simulink model "SimCoJLinkExample_G071"  (R2020b)
settings: Solver=FixedStepDiscrete  StartTime=0.0  StopTime=inf  RelTol=1e-3
undefined symbols (not defined in the file): Cortex, M4
libraries: SimCoJLink x3
settings Model: Creator=beau_  LastModifiedBy=beau_
settings DataIOCC: SaveOutput=off  SignalLogging=off  DSMLogging=off  SaveTime=off  ReturnWorkspaceOutputs=off
settings DebuggingCC: ParameterPrecisionLossMsg=none

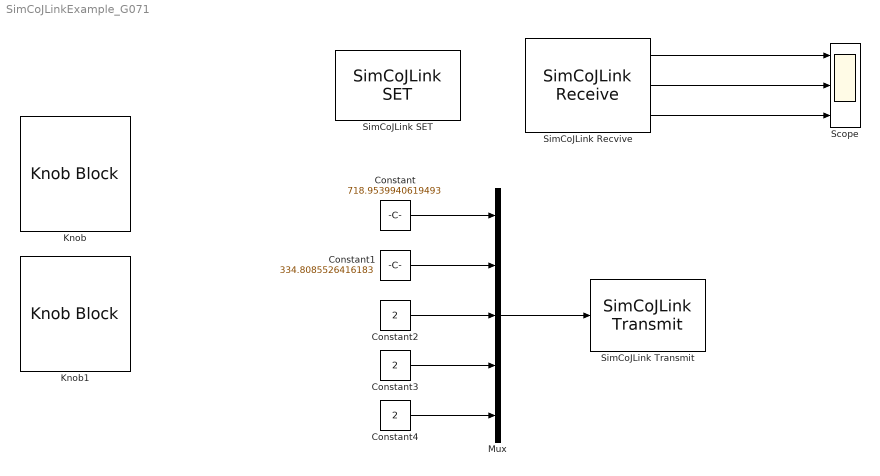
== system SimCoJLinkExample_G071 ==
  Constant : Constant  Value=718.9539940619493  OutDataTypeStr=uint16  SampleTime=0.1
  Constant1 : Constant  Value=334.8085526416183  OutDataTypeStr=uint16  SampleTime=0.1
  Constant2 : Constant  Value=2  OutDataTypeStr=uint16  SampleTime=0.1
  Constant3 : Constant  Value=2  OutDataTypeStr=uint16  SampleTime=0.1
  Constant4 : Constant  Value=2  OutDataTypeStr=uint16  SampleTime=0.1
  Knob : KnobBlock  ScaleMin=100  ScaleMax=4000
  Knob1 : KnobBlock  ScaleMin=100  ScaleMax=2000
  Mux : Mux  Inputs=5
  Scope : Scope  NumInputPorts=3
  SimCoJLink Recvive : SimCoJLink/SimCoJLink Receive  Terminator="\"ET!\""  DataType=uint16  DataSize=[3 1000]  SampleTime=0.1
  SimCoJLink SET : SimCoJLink/SimCoJLink SET  Interface=SWD  Address=0X20000000  AddrLength=0X1000  Speed=50000  Device=Cortex-M4
  SimCoJLink Transmit : SimCoJLink/SimCoJLink Transmit  SampleTime=-1
  wires:
  Mux/1 -> SimCoJLink Transmit/1
  Constant/1 -> Mux/1
  Constant1/1 -> Mux/2
  Constant2/1 -> Mux/3
  Constant3/1 -> Mux/4
  Constant4/1 -> Mux/5
  SimCoJLink Recvive/1 -> Scope/1
  SimCoJLink Recvive/2 -> Scope/2
  SimCoJLink Recvive/3 -> Scope/3
